simulink model "adarbha_hw5_sim"  (Simulink 7.7)
settings: Solver=ode45  StartTime=0.0  StopTime=max(time_s)  RelTol=1e-3
InitFcn:
  | hw5_adarbha
values from neighbouring files (symbols this model uses):
  Area = 2.7    [hw5_adarbha.m]
  Cd = 0.44    [hw5_adarbha.m]
  density = 1.224    [hw5_adarbha.m]
  h_cg_m = 0.45    [hw5_adarbha.m]
  L_a_m = 1.04    [hw5_adarbha.m]
  L_m = 3.04    [hw5_adarbha.m]
  mu = 0.8    [hw5_adarbha.m]
  radius_wheel_m = 0.41    [hw5_adarbha.m]
  rpm = 1:5000    [hw5_adarbha.m]
  Time = xlsread('Malibu_20100929_highway_Baseline','A:A')    [hw5_adarbha.m]
  time_s = time_scale*100    [hw5_adarbha.m]
  vel_m_s = M_number*3    [hw5_adarbha.m]
  Velocity_kph = xlsread('Malibu_20100929_Highway_HW_9_10_2012','B:B')    [hw5_adarbha.m]
  weight_N = 16000    [hw5_adarbha.m]
undefined symbols (not defined in the file or in its folder): torque
libraries: simulink x1
settings Model: Creator=Arjun  LastModifiedBy=Arjun

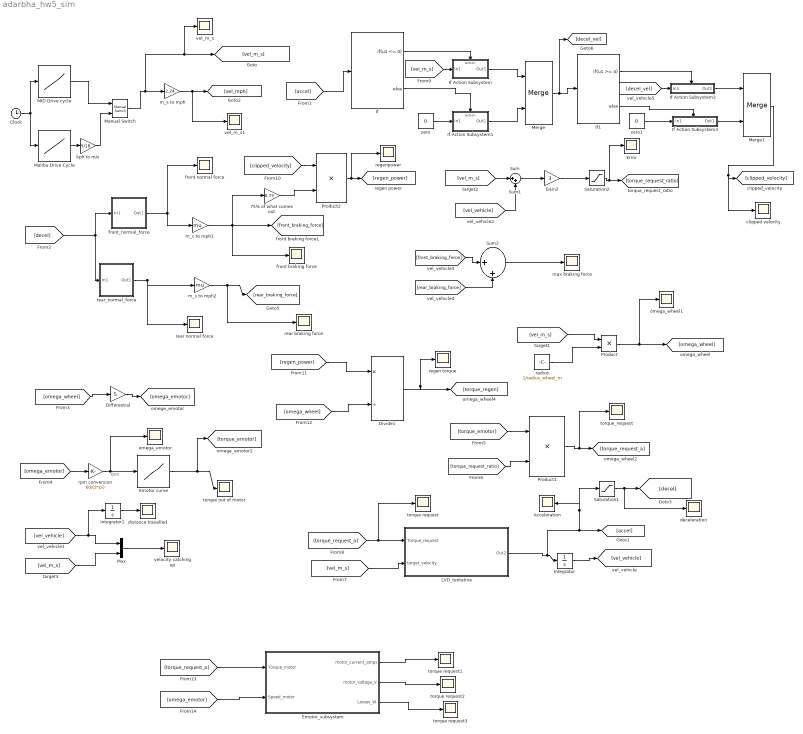
== system adarbha_hw5_sim ==
  note: rpm
  75% of what comes out : Gain  Gain=0.75
  Acceleration : Scope
      settings: SaveName=ScopeData11
  Clock : Clock
      settings: Decimation=10
  Differential : Gain  Gain=5
  Divide1 : Product  Inputs=*/
  Emotor curve : Lookup_n-D  NumberOfTableDimensions=1  BreakpointsForDimension1=rpm  Table=torque  RndMeth=Simplest  InputSameDT=on
  Emotor_subsystem : Subsystem
  Error : Scope
      settings: SaveName=ScopeData17
  Gain2 : Gain  Gain=3
  If : If  IfExpression=u1 <= 0
  If Action Subsystem : Subsystem  TreatAsAtomicUnit=on
  If Action Subsystem1 : Subsystem  TreatAsAtomicUnit=on
  If Action Subsystem2 : Subsystem  TreatAsAtomicUnit=on
  If Action Subsystem3 : Subsystem  TreatAsAtomicUnit=on
  If1 : If  IfExpression=u1 >= 4
  Integrator : Integrator
  Integrator1 : Integrator
  LVD_tentative : Subsystem
  MID Drive cycle : Lookup_n-D  NumberOfTableDimensions=1  BreakpointsForDimension1=time_s  Table=vel_m_s  RndMeth=Simplest  InputSameDT=on
  Malibu Drive Cycle : Lookup_n-D  NumberOfTableDimensions=1  BreakpointsForDimension1=Time  Table=Velocity_kph  RndMeth=Simplest  InputSameDT=on
  Manual Switch : simulink/Signal Routing/Manual Switch  SystemSampleTime=-1  sw=0  action=0  varsize=off
  Merge : Merge
  Merge1 : Merge
  Mux : Mux  Inputs=2
  Product : Product  RndMeth=Zero
  Product1 : Product  RndMeth=Zero
  Product2 : Product  RndMeth=Zero
  Saturation1 : Saturate  UpperLimit=0  LowerLimit=-100
  Saturation2 : Saturate  UpperLimit=1  LowerLimit=-1
  Sum : Sum  Inputs=|+-
  Sum1 : Sum  Inputs=|++
  Sum2 : Sum  Inputs=|++
  clipped velocity : Scope
  deceleration : Scope
  distance travelled : Scope
      settings: SaveName=ScopeData25
  front braking force : Scope
      settings: SaveName=ScopeData16
  front normal force : Scope
      settings: SaveName=ScopeData3
  front_normal_force : Subsystem
  kph to m/s : Gain  Gain=5/18
  m_s to mph : Gain  Gain=2.24
  m_s to mph1 : Gain  Gain=mu
  m_s to mph2 : Gain  Gain=mu
  max braking force : Scope
      settings: SaveName=ScopeData2
  omega_emotor : Scope
      settings: SaveName=ScopeData7
  omega_wheel1 : Scope
      settings: SaveName=ScopeData4
  radius : Constant  Value=1/radius_wheel_m
  rear braking force : Scope
      settings: SaveName=ScopeData19
  rear normal force : Scope
      settings: SaveName=ScopeData5
  rear_normal_force : Subsystem
  regen torque : Scope
      settings: SaveName=ScopeData23
  regenpower : Scope
      settings: SaveName=ScopeData20
  rpm conversion : Gain  Gain=60/(2*pi)
  torque out of motor : Scope
      settings: SaveName=ScopeData8
  torque request{,1..3} (4 alike) : Scope
      torque request settings: SaveName=ScopeData12
      torque request1 settings: SaveName=ScopeData24
      torque request2 settings: SaveName=ScopeData26
      torque request3 settings: SaveName=ScopeData27
  torque_request : Scope
      settings: SaveName=ScopeData6
  vel_m_s : Scope
      settings: SaveName=ScopeData21
  vel_m_s1 : Scope
      settings: YMin=0  YMax=40  SaveName=ScopeData28
  velocity catching up : Scope
      settings: TimeRange=765.8724058416602  YMin=-1e+049  YMax=9.000000000000001e+049  SaveName=ScopeData18
  zero : Constant  Value=0
  zero1 : Constant  Value=0
  wires:
  m_s to mph/1 -> [vel_mph], vel_m_s1/1
  Clock/1 -> MID Drive cycle/1, Malibu Drive Cycle/1
  [decel] -> front_normal_force/1(In1), rear_normal_force/1(In1)
  front_normal_force/1(Out1) -> front normal force/1, m_s to mph1/1
  rear_normal_force/1(Out1) -> rear normal force/1, m_s to mph2/1
  m_s to mph1/1 -> [front_braking_force], front braking force/1, 75% of what comes out/1
  [vel_m_s] -> Product/1
  Product/1 -> [omega_wheel], omega_wheel1/1
  radius/1 -> Product/2
  [torque_emotor] -> Product1/1
  [torque_request_ratio] -> Product1/2
  Product1/1 -> [torque_request_a], torque_request/1
  [omega_wheel] -> Differential/1
  Differential/1 -> [omega_emotor]
  [omega_emotor] -> rpm conversion/1
  rpm conversion/1 -> Emotor curve/1, omega_emotor/1
  Emotor curve/1 -> torque out of motor/1, [torque_emotor]
  [vel_m_s] -> LVD_tentative/2(target_velocity)
  [torque_request_a] -> LVD_tentative/1(Torque_request), torque request/1
  Integrator/1 -> [vel_vehicle]
  LVD_tentative/1(Out2) -> Integrator/1, [accel], Saturation1/1, Acceleration/1
  [vel_m_s] -> Sum/1
  [vel_vehicle] -> Sum/2
  [vel_m_s] -> Mux/2
  [vel_vehicle] -> Mux/1, Integrator1/1
  Mux/1 -> velocity catching up/1
  m_s to mph2/1 -> [rear_braking_force], rear braking force/1
  [front_braking_force] -> Sum2/1
  [rear_braking_force] -> Sum2/2
  Sum2/1 -> max braking force/1
  Saturation1/1 -> [decel], deceleration/1
  [accel] -> If/1
  If/1 -> If Action Subsystem/Action
  [vel_m_s] -> If Action Subsystem/1(In1)
  If/2 -> If Action Subsystem1/Action
  zero/1 -> If Action Subsystem1/1(In1)
  If Action Subsystem/1(Out1) -> Merge/1
  If Action Subsystem1/1(Out1) -> Merge/2
  75% of what comes out/1 -> Product2/2
  [clipped_velocity] -> Product2/1
  Product2/1 -> [regen_power], regenpower/1
  Merge/1 -> If1/1, [decel_vel]
  If1/1 -> If Action Subsystem2/Action
  If1/2 -> If Action Subsystem3/Action
  [decel_vel] -> If Action Subsystem2/1(In1)
  zero1/1 -> If Action Subsystem3/1(In1)
  If Action Subsystem2/1(Out1) -> Merge1/1
  If Action Subsystem3/1(Out1) -> Merge1/2
  Merge1/1 -> clipped velocity/1, [clipped_velocity]
  [regen_power] -> Divide1/1
  [omega_wheel] -> Divide1/2
  Divide1/1 -> regen torque/1, [torque_regen]
  MID Drive cycle/1 -> Manual Switch/1
  Manual Switch/1 -> m_s to mph/1, [vel_m_s], vel_m_s/1
  Malibu Drive Cycle/1 -> kph to m/s/1
  kph to m/s/1 -> Manual Switch/2
  Integrator1/1 -> distance travelled/1
  [torque_request_a] -> Emotor_subsystem/1(Torque_motor)
  [omega_emotor] -> Emotor_subsystem/2(Speed_motor)
  Emotor_subsystem/1(motor_current_amps) -> torque request1/1
  Emotor_subsystem/2(motor_voltage_V) -> torque request2/1
  Emotor_subsystem/3(Losses_W) -> torque request3/1
  Saturation2/1 -> [torque_request_ratio], Error/1
  Gain2/1 -> Saturation2/1
  Sum/1 -> Gain2/1

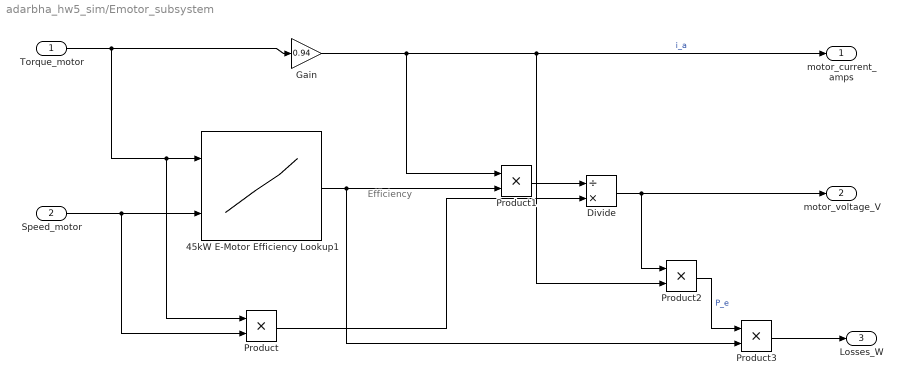
== system adarbha_hw5_sim/Emotor_subsystem ==
  note: Efficiency
  Torque_motor : Inport
  Speed_motor : Inport  Port=2
  45kW E-Motor Efficiency Lookup1 : Lookup2D  RowIndex=[0,50,100,150,200,250,300,350,400,400,500,550]  ColumnIndex=[0,500,1000,1500,2000,2050,3000,3500,4000,4500]  Table=reshape([0.5,0.7,0.73,0.72,0.72,0.69,0.68,0.67,0.62,0.6,0.55,0.5,0.5,0.7,0.81,0.82,0.82,0.82,0.81,0.8,0.78,0.78,0.76,0.75,0.5,0.78,0.85,0.865,0.88,0.88,0.865,0.875,0.87,0.86,0.855,0.85,0.5,0.73,0.865,0.88,0.9,0.9,0.905,0.905,0.9,0.89,0.895,0.88,0.5,0.7,0.875,0.905,0.91,0.91,0.915,0.915,0.92,0.925,.925,0,0.5,0.8,0.875,0.905,0.915,0.92,0.92,0.925,0.93,0.93,0,0,0.5,0.76,0.875,0.9,0.925,0.94,0.95,0.96,0,0,0,0,0.5,0.76,0.875,0.9,0.925,0.935,0.935,0,0,0,0,0,0.5,0.75,0.87,0.905,0.925,0.925,0,0,0,0,0,0,0.5,0.75,0.865,0.905,0.92,0.92,0,0,0,0,0,0],12,10)
  Divide : Product  Inputs=/*
  Gain : Gain  Gain=0.94
  Product{,1..3} (4 alike) : Product  RndMeth=Zero
  motor_current_amps : Outport
  motor_voltage_V : Outport  Port=2
  Losses_W : Outport  Port=3
  wires:
  Torque_motor/1 -> Gain/1, 45kW E-Motor Efficiency Lookup1/1, Product/1
  Speed_motor/1 -> 45kW E-Motor Efficiency Lookup1/2, Product/2
  Gain/1 -> Product1/1, motor_current_amps/1, Product2/2  "i_a"
  45kW E-Motor Efficiency Lookup1/1 -> Product1/2, Product3/2
  Product1/1 -> Divide/1
  Product/1 -> Divide/2
  Divide/1 -> motor_voltage_V/1, Product2/1
  Product2/1 -> Product3/1  "P_e"
  Product3/1 -> Losses_W/1

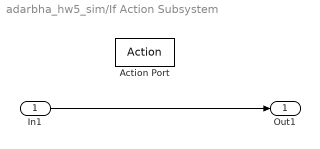
== system adarbha_hw5_sim/If Action Subsystem ==
  In1 : Inport
  Action Port : ActionPort  ActionType=then
  Out1 : Outport
  wires:
  In1/1 -> Out1/1

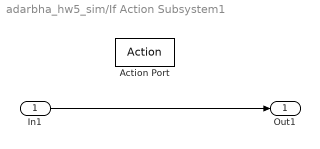
== system adarbha_hw5_sim/If Action Subsystem1 ==
  In1 : Inport
  Action Port : ActionPort  ActionType=else
  Out1 : Outport
  wires:
  In1/1 -> Out1/1

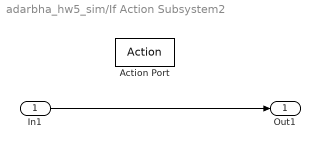
== system adarbha_hw5_sim/If Action Subsystem2 ==
  In1 : Inport
  Action Port : ActionPort  ActionType=then
  Out1 : Outport
  wires:
  In1/1 -> Out1/1

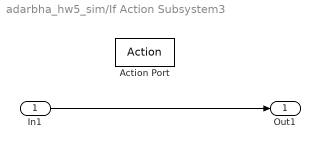
== system adarbha_hw5_sim/If Action Subsystem3 ==
  In1 : Inport
  Action Port : ActionPort  ActionType=else
  Out1 : Outport
  wires:
  In1/1 -> Out1/1

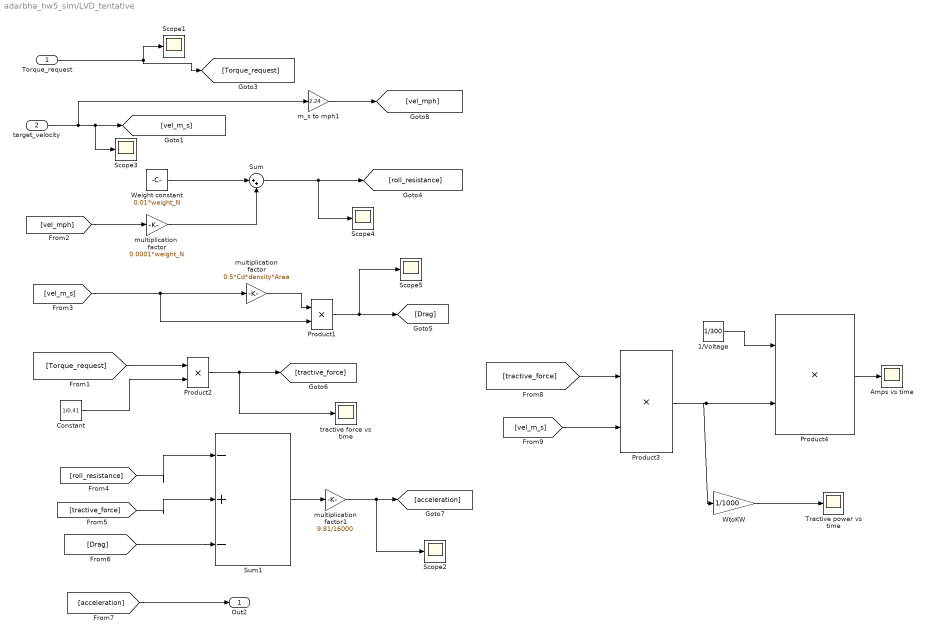
== system adarbha_hw5_sim/LVD_tentative ==
  Torque_request : Inport
  target_velocity : Inport  Port=2
  1/Voltage : Constant  Value=1/300
  Amps vs time : Scope
      settings: SaveName=ScopeData15
  Constant : Constant  Value=1/0.41
  Product{1..4} (4 alike) : Product  RndMeth=Zero
  Scope{1..5} (5 alike) : Scope
      Scope1 settings: SaveName=ScopeData5
      Scope2 settings: SaveName=ScopeData6
      Scope3 settings: SaveName=ScopeData8
      Scope4 settings: SaveName=ScopeData9
      Scope5 settings: SaveName=ScopeData10
  Sum : Sum  Inputs=|++
  Sum1 : Sum  Inputs=|-+-
  Tractive power vs time : Scope
      settings: SaveName=ScopeData14
  Weight constant : Constant  Value=0.01*weight_N
  WtoKW : Gain  Gain=1/1000
  m_s to mph1 : Gain  Gain=2.24
  multiplication  factor : Gain  Gain=0.0001*weight_N
  multiplication factor : Gain  Gain=0.5*Cd*density*Area
  multiplication factor1 : Gain  Gain=9.81/16000
  tractive force vs time : Scope
      settings: SaveName=ScopeData13
  Out2 : Outport
  wires:
  Weight constant/1 -> Sum/1
  multiplication  factor/1 -> Sum/2
  Sum/1 -> [roll_resistance], Scope4/1
  [vel_mph] -> multiplication  factor/1
  multiplication factor/1 -> Product1/1
  [vel_m_s] -> multiplication factor/1, Product1/2
  Product1/1 -> [Drag], Scope5/1
  [Torque_request] -> Product2/1
  Constant/1 -> Product2/2
  Product2/1 -> [tractive_force], tractive force vs time/1
  [roll_resistance] -> Sum1/1
  [tractive_force] -> Sum1/2
  [Drag] -> Sum1/3
  Sum1/1 -> multiplication factor1/1
  multiplication factor1/1 -> [acceleration], Scope2/1
  Torque_request/1 -> [Torque_request], Scope1/1
  target_velocity/1 -> m_s to mph1/1, [vel_m_s], Scope3/1
  m_s to mph1/1 -> [vel_mph]
  [acceleration] -> Out2/1
  [tractive_force] -> Product3/1
  [vel_m_s] -> Product3/2
  Product3/1 -> Product4/2, WtoKW/1
  1/Voltage/1 -> Product4/1
  Product4/1 -> Amps vs time/1
  WtoKW/1 -> Tractive power vs time/1

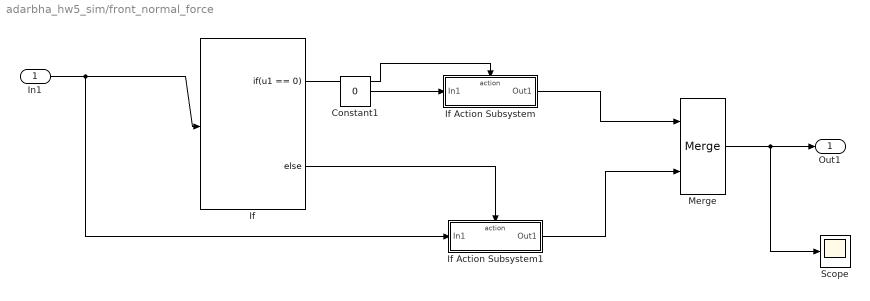
== system adarbha_hw5_sim/front_normal_force ==
  In1 : Inport
  Constant1 : Constant  Value=0
  If : If  IfExpression=u1 == 0
  If Action Subsystem : Subsystem  TreatAsAtomicUnit=on
  If Action Subsystem1 : Subsystem  TreatAsAtomicUnit=on
  Merge : Merge
  Scope : Scope
      settings: SaveName=ScopeData22
  Out1 : Outport
  wires:
  In1/1 -> If/1, If Action Subsystem1/1(In1)
  If/1 -> If Action Subsystem/Action
  Constant1/1 -> If Action Subsystem/1(In1)
  Merge/1 -> Out1/1, Scope/1
  If Action Subsystem/1(Out1) -> Merge/1
  If/2 -> If Action Subsystem1/Action
  If Action Subsystem1/1(Out1) -> Merge/2

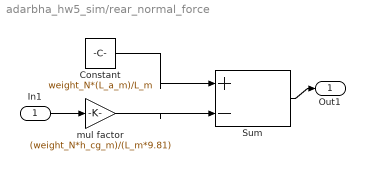
== system adarbha_hw5_sim/rear_normal_force ==
  In1 : Inport
  Constant : Constant  Value=weight_N*(L_a_m)/L_m
  Sum : Sum  Inputs=|+-
  mul factor : Gain  Gain=(weight_N*h_cg_m)/(L_m*9.81)
  Out1 : Outport
  wires:
  mul factor/1 -> Sum/2
  Constant/1 -> Sum/1
  In1/1 -> mul factor/1
  Sum/1 -> Out1/1

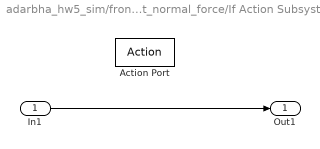
== system adarbha_hw5_sim/front_normal_force/If Action Subsystem ==
  In1 : Inport
  Action Port : ActionPort  ActionType=then
  Out1 : Outport
  wires:
  In1/1 -> Out1/1

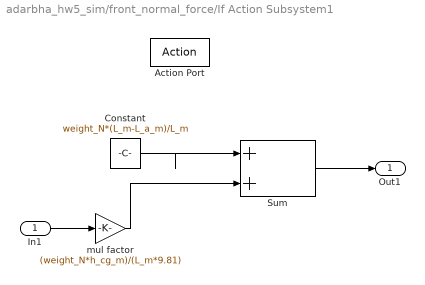
== system adarbha_hw5_sim/front_normal_force/If Action Subsystem1 ==
  In1 : Inport
  Action Port : ActionPort  ActionType=else
  Constant : Constant  Value=weight_N*(L_m-L_a_m)/L_m
  Sum : Sum  Inputs=|++
  mul factor : Gain  Gain=(weight_N*h_cg_m)/(L_m*9.81)
  Out1 : Outport
  wires:
  mul factor/1 -> Sum/2
  Constant/1 -> Sum/1
  In1/1 -> mul factor/1
  Sum/1 -> Out1/1
